simulink library "CommercialVehicleLibrary2G"  (R2021a)
settings: Solver=VariableStepAuto  StartTime=0.0  StopTime=10.0  RelTol=1e-3
values from neighbouring files (symbols this model uses):
  brake_input = [0   tmax ... (first row only)    [init_vehicle.m]    (also in run_Circle.m = [0  tmax; run_Coastdown.m = [0  2  tmax; run_DoubleLaneChangeDriver.m = [0   2  tmax; run_MaxAcc.m = [0  2  tmax)
  pose_t0 = [0 0 0 0]    [init_vehicle.m]    (also in run_Circle.m; run_Coastdown.m; run_DoubleLaneChangeDriver.m; run_MaxAcc.m)
  rdfname = 'TNO_FlatRoad.rdf'    [run_Circle.m]    (also in run_Coastdown.m; run_DoubleLaneChangeDriver.m; run_MaxAcc.m; run_Rollover.m)
  rdfname_inner = 'TNO_FlatRoad.rdf'    [run_Circle.m]    (also in run_Coastdown.m; run_DoubleLaneChangeDriver.m; run_MaxAcc.m; run_Rollover.m)
  steer_input = [0  tmax ... (first row only)    [init_vehicle.m]    (also in run_Circle.m = [0  2   10     13       tmax; run_Coastdown.m = [0 tmax; run_DoubleLaneChangeDriver.m = [0 tmax; run_MaxAcc.m = [0 tmax)
  throttle_input = [0         tmax ... (first row only)    [init_vehicle.m]    (also in run_Circle.m; run_Coastdown.m = [0        10         10.0001 tmax; run_DoubleLaneChangeDriver.m = [0        tmax; run_MaxAcc.m = [0        tmax)
  Vx = 0    [init_vehicle.m]    (also in run_Circle.m = Vx_kmh/3.6; run_Coastdown.m = Vx_kmh/3.6; run_DoubleLaneChangeDriver.m = Vx_kmh/3.6; run_MaxAcc.m)
  Vx_input = [0  tmax ... (first row only)    [init_vehicle.m]    (also in run_Circle.m; run_Coastdown.m = [0 tmax; run_DoubleLaneChangeDriver.m = [0 tmax; run_MaxAcc.m = [0 tmax)
undefined symbols (not defined in the file or in its folder): Drive, Floor, Fzstat, Fzstat1, Fzstat3, l, l_load1, l_load2, lbar, mass_load1, mass_load2, psi_semitrailer, rho, rim_Ixx, rim_Iyy, rim_mass, Steer, steer_path, tpfname, X, x_torsion, xcg, xcg1, xcg2, xcg_front, xcg_rear, xdrive1, xload1, xload2, xpos1, xref, xrev1, Xt0, Y, Yt0, Z
libraries: sm_lib x291, $bdroot x157, nesl_utility x143, vrlib x1
(part 11 of 12)

== system CommercialVehicleLibrary2G/Components/MF Tyre L/add signal names2 ==
  In1 : Inport
  Bus Creator : BusCreator  Inputs=40
  Bus Creator1 : BusCreator  Inputs=20
  Demux1 : Demux  Outputs=60
      settings: DisplayOption=none
  Terminator : Terminator
  varinf : Outport
  wires:
  Bus Creator1/1 -> Terminator/1
  Demux1/60 -> Bus Creator1/20
  Demux1/59 -> Bus Creator1/19
  Demux1/58 -> Bus Creator1/18
  Demux1/57 -> Bus Creator1/17
  Demux1/56 -> Bus Creator1/16
  Demux1/55 -> Bus Creator1/15
  Demux1/54 -> Bus Creator1/14
  Demux1/53 -> Bus Creator1/13
  Demux1/52 -> Bus Creator1/12
  Demux1/51 -> Bus Creator1/11
  Demux1/50 -> Bus Creator1/10
  Demux1/49 -> Bus Creator1/9
  Demux1/48 -> Bus Creator1/8
  Demux1/47 -> Bus Creator1/7
  Demux1/46 -> Bus Creator1/6
  Demux1/45 -> Bus Creator1/5
  Demux1/44 -> Bus Creator1/4
  Demux1/43 -> Bus Creator1/3
  Demux1/42 -> Bus Creator1/2
  Demux1/41 -> Bus Creator1/1
  Demux1/39 -> Bus Creator/39  "eff_plane_curvature"
  Demux1/38 -> Bus Creator/38  "eff_plane_angle"
  Demux1/37 -> Bus Creator/37  "eff_plane_height"
  Demux1/36 -> Bus Creator/36  "nz"
  Demux1/35 -> Bus Creator/35  "ny"
  Demux1/34 -> Bus Creator/34  "nx"
  Demux1/33 -> Bus Creator/33  "zcp"
  Demux1/32 -> Bus Creator/32  "ycp"
  Demux1/31 -> Bus Creator/31  "xcp"
  Demux1/30 -> Bus Creator/30  "_e30"
  Demux1/29 -> Bus Creator/29  "_e29"
  Demux1/28 -> Bus Creator/28  "travelled_distance"
  Demux1/27 -> Bus Creator/27  "_e27"
  Demux1/26 -> Bus Creator/26  "_e26"
  Demux1/25 -> Bus Creator/25  "_e25"
  Demux1/24 -> Bus Creator/24  "psidot"
  Demux1/23 -> Bus Creator/23  "Vz"
  Demux1/40 -> Bus Creator/40  "eff_plane_banking"
  Demux1/22 -> Bus Creator/22  "Vsy"
  Demux1/21 -> Bus Creator/21  "Vsx"
  Demux1/20 -> Bus Creator/20  "relaxation_length_y"
  Demux1/19 -> Bus Creator/19  "relaxation_length_x"
  Demux1/18 -> Bus Creator/18  "mu_y"
  Demux1/17 -> Bus Creator/17  "mu_x"
  Demux1/16 -> Bus Creator/16  "pneumatic_trail"
  Demux1/15 -> Bus Creator/15  "contact_length"
  Demux1/14 -> Bus Creator/14  "vertical_deflection"
  Demux1/13 -> Bus Creator/13  "effective_rolling_radius"
  Demux1/12 -> Bus Creator/12  "_e12"
  Demux1/11 -> Bus Creator/11  "Vx"
  Demux1/10 -> Bus Creator/10  "turn_slip"
  Demux1/9 -> Bus Creator/9  "inclination_angle"
  Demux1/8 -> Bus Creator/8  "side_slip_angle"
  Demux1/7 -> Bus Creator/7  "longitudinal_slip"
  Demux1/6 -> Bus Creator/6  "Mz"
  Demux1/5 -> Bus Creator/5  "My"
  Demux1/4 -> Bus Creator/4  "Mx"
  Demux1/3 -> Bus Creator/3  "Fz"
  Demux1/2 -> Bus Creator/2  "Fy"
  Demux1/1 -> Bus Creator/1  "Fx"
  In1/1 -> Demux1/1
  Bus Creator/1 -> varinf/1  "varinf"

== system CommercialVehicleLibrary2G/Components/MF Tyre R/add signal names2 ==
  In1 : Inport
  Bus Creator : BusCreator  Inputs=40
  Bus Creator1 : BusCreator  Inputs=20
  Demux1 : Demux  Outputs=60
      settings: DisplayOption=none
  Terminator : Terminator
  varinf : Outport
  wires:
  Bus Creator1/1 -> Terminator/1
  Demux1/60 -> Bus Creator1/20
  Demux1/59 -> Bus Creator1/19
  Demux1/58 -> Bus Creator1/18
  Demux1/57 -> Bus Creator1/17
  Demux1/56 -> Bus Creator1/16
  Demux1/55 -> Bus Creator1/15
  Demux1/54 -> Bus Creator1/14
  Demux1/53 -> Bus Creator1/13
  Demux1/52 -> Bus Creator1/12
  Demux1/51 -> Bus Creator1/11
  Demux1/50 -> Bus Creator1/10
  Demux1/49 -> Bus Creator1/9
  Demux1/48 -> Bus Creator1/8
  Demux1/47 -> Bus Creator1/7
  Demux1/46 -> Bus Creator1/6
  Demux1/45 -> Bus Creator1/5
  Demux1/44 -> Bus Creator1/4
  Demux1/43 -> Bus Creator1/3
  Demux1/42 -> Bus Creator1/2
  Demux1/41 -> Bus Creator1/1
  Demux1/39 -> Bus Creator/39  "eff_plane_curvature"
  Demux1/38 -> Bus Creator/38  "eff_plane_angle"
  Demux1/37 -> Bus Creator/37  "eff_plane_height"
  Demux1/36 -> Bus Creator/36  "nz"
  Demux1/35 -> Bus Creator/35  "ny"
  Demux1/34 -> Bus Creator/34  "nx"
  Demux1/33 -> Bus Creator/33  "zcp"
  Demux1/32 -> Bus Creator/32  "ycp"
  Demux1/31 -> Bus Creator/31  "xcp"
  Demux1/30 -> Bus Creator/30  "_e30"
  Demux1/29 -> Bus Creator/29  "_e29"
  Demux1/28 -> Bus Creator/28  "travelled_distance"
  Demux1/27 -> Bus Creator/27  "_e27"
  Demux1/26 -> Bus Creator/26  "_e26"
  Demux1/25 -> Bus Creator/25  "_e25"
  Demux1/24 -> Bus Creator/24  "psidot"
  Demux1/23 -> Bus Creator/23  "Vz"
  Demux1/40 -> Bus Creator/40  "eff_plane_banking"
  Demux1/22 -> Bus Creator/22  "Vsy"
  Demux1/21 -> Bus Creator/21  "Vsx"
  Demux1/20 -> Bus Creator/20  "relaxation_length_y"
  Demux1/19 -> Bus Creator/19  "relaxation_length_x"
  Demux1/18 -> Bus Creator/18  "mu_y"
  Demux1/17 -> Bus Creator/17  "mu_x"
  Demux1/16 -> Bus Creator/16  "pneumatic_trail"
  Demux1/15 -> Bus Creator/15  "contact_length"
  Demux1/14 -> Bus Creator/14  "vertical_deflection"
  Demux1/13 -> Bus Creator/13  "effective_rolling_radius"
  Demux1/12 -> Bus Creator/12  "_e12"
  Demux1/11 -> Bus Creator/11  "Vx"
  Demux1/10 -> Bus Creator/10  "turn_slip"
  Demux1/9 -> Bus Creator/9  "inclination_angle"
  Demux1/8 -> Bus Creator/8  "side_slip_angle"
  Demux1/7 -> Bus Creator/7  "longitudinal_slip"
  Demux1/6 -> Bus Creator/6  "Mz"
  Demux1/5 -> Bus Creator/5  "My"
  Demux1/4 -> Bus Creator/4  "Mx"
  Demux1/3 -> Bus Creator/3  "Fz"
  Demux1/2 -> Bus Creator/2  "Fy"
  Demux1/1 -> Bus Creator/1  "Fx"
  In1/1 -> Demux1/1
  Bus Creator/1 -> varinf/1  "varinf"

== system CommercialVehicleLibrary2G/Trailers/Semitrailer/Cameras ==
  Spherical Solid : sm_lib/Body Elements/Spherical Solid  GraphicAmbientColor=[0.15 0.15 0.15 1.0]  BasedOnType=Density  CenterOfMass=[0 0 0]  CenterOfMassUnits=m  GraphicDiffuseColor=[0.5 0.5 0.5]  Density=1000  DensityUnits=kg/m^3  DoExposeReferenceFrame=on  GraphicEmissiveColor=[0.0 0.0 0.0 1.0]  ExportEntireGeometry=off  SerializedExposedGeometries=<ExposedGeometries/>  SerializedFrames=<Frames/>  MarkerShape=Sphere  MarkerSize=10  GraphicType=FromGeometry  InertiaType=PointMass  Mass=1e-10  MassUnits=kg  MomentsOfInertia=[1 1 1]  MomentsOfInertiaUnits=kg*m^2  GraphicOpacity=0  ProductsOfInertia=[0 0 0]  ProductsOfInertiaUnits=kg*m^2  GraphicShininess=75  GraphicSpecularColor=[0.5 0.5 0.5 1.0]  SphereRadius=1e-10  SphereRadiusUnits=m  GraphicVisPropType=SimpleVisualProperties
  Trailer Camera Position : sm_lib/Frames and Transforms/Rigid Transform  TranslationMethod=Cartesian  TranslationStandardOffset=0  TranslationLengthUnit=m  TranslationStandardAxis=+Z  TranslationCartesianOffset=[-20 0 8]  TranslationROffset=0  TranslationROffsetUnits=m  TranslationZOffset=0  TranslationZOffsetUnits=m  TranslationThetaOffset=0  TranslationThetaOffsetUnits=deg  RotationMethod=None  RotationAngleUnits=deg  RotationStandardAxis=+Z  RotationAngle=0.0  RotationArbitraryAxis=[0 0 1]  FollAlignAxisA=+X  BaseAlignAxisA=+Y  FollAlignAxisB=+Y  BaseAlignAxisB=+Z  RotationSequenceAxes=FollowerAxes  RotationSequence=XYX  RotationSequenceAngles=[0 0 0]  RotationSequenceAnglesUnits=deg  RotationMatrix=[1 0 0; 0 1 0; 0 0 1]
  " " : PMIOPort  Side=Right
  connections:
  Spherical Solid/RConn1 -- Trailer Camera Position/RConn1
  Trailer Camera Position/LConn1 -- " "/RConn1

== system CommercialVehicleLibrary2G/Trailers/Trailer - 2 axle /Cameras ==
  Spherical Solid : sm_lib/Body Elements/Spherical Solid  GraphicAmbientColor=[0.15 0.15 0.15 1.0]  BasedOnType=Density  CenterOfMass=[0 0 0]  CenterOfMassUnits=m  GraphicDiffuseColor=[0.5 0.5 0.5]  Density=1000  DensityUnits=kg/m^3  DoExposeReferenceFrame=on  GraphicEmissiveColor=[0.0 0.0 0.0 1.0]  ExportEntireGeometry=off  SerializedExposedGeometries=<ExposedGeometries/>  SerializedFrames=<Frames/>  MarkerShape=Sphere  MarkerSize=10  GraphicType=FromGeometry  InertiaType=PointMass  Mass=1e-10  MassUnits=kg  MomentsOfInertia=[1 1 1]  MomentsOfInertiaUnits=kg*m^2  GraphicOpacity=0  ProductsOfInertia=[0 0 0]  ProductsOfInertiaUnits=kg*m^2  GraphicShininess=75  GraphicSpecularColor=[0.5 0.5 0.5 1.0]  SphereRadius=1e-10  SphereRadiusUnits=m  GraphicVisPropType=SimpleVisualProperties
  Trailer Camera Position : sm_lib/Frames and Transforms/Rigid Transform  TranslationMethod=Cartesian  TranslationStandardOffset=0  TranslationLengthUnit=m  TranslationStandardAxis=+Z  TranslationCartesianOffset=[-20 0 8]  TranslationROffset=0  TranslationROffsetUnits=m  TranslationZOffset=0  TranslationZOffsetUnits=m  TranslationThetaOffset=0  TranslationThetaOffsetUnits=deg  RotationMethod=None  RotationAngleUnits=deg  RotationStandardAxis=+Z  RotationAngle=0.0  RotationArbitraryAxis=[0 0 1]  FollAlignAxisA=+X  BaseAlignAxisA=+Y  FollAlignAxisB=+Y  BaseAlignAxisB=+Z  RotationSequenceAxes=FollowerAxes  RotationSequence=XYX  RotationSequenceAngles=[0 0 0]  RotationSequenceAnglesUnits=deg  RotationMatrix=[1 0 0; 0 1 0; 0 0 1]
  " " : PMIOPort  Side=Right
  connections:
  Spherical Solid/RConn1 -- Trailer Camera Position/RConn1
  Trailer Camera Position/LConn1 -- " "/RConn1

== system CommercialVehicleLibrary2G/Trailers/Trailer - 3 axle /Cameras ==
  Spherical Solid : sm_lib/Body Elements/Spherical Solid  GraphicAmbientColor=[0.15 0.15 0.15 1.0]  BasedOnType=Density  CenterOfMass=[0 0 0]  CenterOfMassUnits=m  GraphicDiffuseColor=[0.5 0.5 0.5]  Density=1000  DensityUnits=kg/m^3  DoExposeReferenceFrame=on  GraphicEmissiveColor=[0.0 0.0 0.0 1.0]  ExportEntireGeometry=off  SerializedExposedGeometries=<ExposedGeometries/>  SerializedFrames=<Frames/>  MarkerShape=Sphere  MarkerSize=10  GraphicType=FromGeometry  InertiaType=PointMass  Mass=1e-10  MassUnits=kg  MomentsOfInertia=[1 1 1]  MomentsOfInertiaUnits=kg*m^2  GraphicOpacity=0  ProductsOfInertia=[0 0 0]  ProductsOfInertiaUnits=kg*m^2  GraphicShininess=75  GraphicSpecularColor=[0.5 0.5 0.5 1.0]  SphereRadius=1e-10  SphereRadiusUnits=m  GraphicVisPropType=SimpleVisualProperties
  Trailer Camera Position : sm_lib/Frames and Transforms/Rigid Transform  TranslationMethod=Cartesian  TranslationStandardOffset=0  TranslationLengthUnit=m  TranslationStandardAxis=+Z  TranslationCartesianOffset=[-20 0 8]  TranslationROffset=0  TranslationROffsetUnits=m  TranslationZOffset=0  TranslationZOffsetUnits=m  TranslationThetaOffset=0  TranslationThetaOffsetUnits=deg  RotationMethod=None  RotationAngleUnits=deg  RotationStandardAxis=+Z  RotationAngle=0.0  RotationArbitraryAxis=[0 0 1]  FollAlignAxisA=+X  BaseAlignAxisA=+Y  FollAlignAxisB=+Y  BaseAlignAxisB=+Z  RotationSequenceAxes=FollowerAxes  RotationSequence=XYX  RotationSequenceAngles=[0 0 0]  RotationSequenceAnglesUnits=deg  RotationMatrix=[1 0 0; 0 1 0; 0 0 1]
  " " : PMIOPort  Side=Right
  connections:
  Spherical Solid/RConn1 -- Trailer Camera Position/RConn1
  Trailer Camera Position/LConn1 -- " "/RConn1

== system CommercialVehicleLibrary2G/Utilities/To_workspace_dolly/Subsystem ==
  In1 : Inport
  Bus Selector24 : BusSelector  OutputSignals=axle1.Tire_L.Fx,axle1.Tire_R.Fx,axle2.Tire_L.Fx,axle2.Tire_R.Fx
  Mux : Mux
  Out1 : Outport
  wires:
  Bus Selector24/4 -> Mux/4  "<Fx>"
  Bus Selector24/3 -> Mux/3  "<Fx>"
  Bus Selector24/2 -> Mux/2  "<Fx>"
  Bus Selector24/1 -> Mux/1  "<Fx>"
  Mux/1 -> Out1/1
  In1/1 -> Bus Selector24/1

== system CommercialVehicleLibrary2G/Utilities/To_workspace_dolly/Subsystem1 ==
  In1 : Inport
  Bus Selector24 : BusSelector  OutputSignals=axle1.Tire_L.Fy,axle1.Tire_R.Fy,axle2.Tire_L.Fy,axle2.Tire_R.Fy
  Mux : Mux
  Out1 : Outport
  wires:
  Mux/1 -> Out1/1
  In1/1 -> Bus Selector24/1
  Bus Selector24/1 -> Mux/1  "<Fy>"
  Bus Selector24/2 -> Mux/2  "<Fy>"
  Bus Selector24/3 -> Mux/3  "<Fy>"
  Bus Selector24/4 -> Mux/4  "<Fy>"

== system CommercialVehicleLibrary2G/Utilities/To_workspace_dolly/Subsystem2 ==
  In1 : Inport
  Bus Selector24 : BusSelector  OutputSignals=axle1.Tire_L.Fz,axle1.Tire_R.Fz,axle2.Tire_L.Fz,axle2.Tire_R.Fz
  Mux : Mux
  Out1 : Outport
  wires:
  Mux/1 -> Out1/1
  In1/1 -> Bus Selector24/1
  Bus Selector24/1 -> Mux/1  "<Fz>"
  Bus Selector24/2 -> Mux/2  "<Fz>"
  Bus Selector24/3 -> Mux/3  "<Fz>"
  Bus Selector24/4 -> Mux/4  "<Fz>"

== system CommercialVehicleLibrary2G/Utilities/To_workspace_dolly/Subsystem3 ==
  In1 : Inport
  Bus Selector6 : BusSelector  OutputSignals=axle1.Omega1,axle1.Omega2,axle2.Omega1,axle2.Omega2
  Mux : Mux
  Out1 : Outport
  wires:
  In1/1 -> Bus Selector6/1
  Mux/1 -> Out1/1
  Bus Selector6/1 -> Mux/1  "<Omega1>"
  Bus Selector6/2 -> Mux/2  "<Omega2>"
  Bus Selector6/3 -> Mux/3  "<Omega1>"
  Bus Selector6/4 -> Mux/4  "<Omega2>"

== system CommercialVehicleLibrary2G/Utilities/To_workspace_drawbar_trailer_2axle/Subsystem ==
  In1 : Inport
  Bus Selector24 : BusSelector  OutputSignals=axle1.Tire_L.Fx,axle1.Tire_R.Fx,axle2.Tire_L.Fx,axle2.Tire_R.Fx
  Mux : Mux
  Out1 : Outport
  wires:
  Bus Selector24/4 -> Mux/4  "<Fx>"
  Bus Selector24/3 -> Mux/3  "<Fx>"
  Bus Selector24/2 -> Mux/2  "<Fx>"
  Bus Selector24/1 -> Mux/1  "<Fx>"
  Mux/1 -> Out1/1
  In1/1 -> Bus Selector24/1

== system CommercialVehicleLibrary2G/Utilities/To_workspace_drawbar_trailer_2axle/Subsystem1 ==
  In1 : Inport
  Bus Selector24 : BusSelector  OutputSignals=axle1.Tire_L.Fy,axle1.Tire_R.Fy,axle2.Tire_L.Fy,axle2.Tire_R.Fy
  Mux : Mux
  Out1 : Outport
  wires:
  Mux/1 -> Out1/1
  In1/1 -> Bus Selector24/1
  Bus Selector24/1 -> Mux/1  "<Fy>"
  Bus Selector24/2 -> Mux/2  "<Fy>"
  Bus Selector24/3 -> Mux/3  "<Fy>"
  Bus Selector24/4 -> Mux/4  "<Fy>"

== system CommercialVehicleLibrary2G/Utilities/To_workspace_drawbar_trailer_2axle/Subsystem2 ==
  In1 : Inport
  Bus Selector24 : BusSelector  OutputSignals=axle1.Tire_L.Fz,axle1.Tire_R.Fz,axle2.Tire_L.Fz,axle2.Tire_R.Fz
  Mux : Mux
  Out1 : Outport
  wires:
  Mux/1 -> Out1/1
  In1/1 -> Bus Selector24/1
  Bus Selector24/1 -> Mux/1  "<Fz>"
  Bus Selector24/2 -> Mux/2  "<Fz>"
  Bus Selector24/3 -> Mux/3  "<Fz>"
  Bus Selector24/4 -> Mux/4  "<Fz>"

== system CommercialVehicleLibrary2G/Utilities/To_workspace_drawbar_trailer_2axle/Subsystem3 ==
  In1 : Inport
  Bus Selector6 : BusSelector  OutputSignals=axle1.Omega1,axle1.Omega2,axle2.Omega1,axle2.Omega2
  Mux : Mux
  Out1 : Outport
  wires:
  In1/1 -> Bus Selector6/1
  Mux/1 -> Out1/1
  Bus Selector6/1 -> Mux/1  "<Omega1>"
  Bus Selector6/2 -> Mux/2  "<Omega2>"
  Bus Selector6/3 -> Mux/3  "<Omega1>"
  Bus Selector6/4 -> Mux/4  "<Omega2>"

== system CommercialVehicleLibrary2G/Utilities/To_workspace_drawbar_trailer_3axle/Subsystem ==
  In1 : Inport
  Bus Selector24 : BusSelector  OutputSignals=axle1.Tire_L.Fx,axle1.Tire_R.Fx,axle2.Tire_L.Fx,axle2.Tire_R.Fx
  Mux : Mux
  Out1 : Outport
  wires:
  Bus Selector24/4 -> Mux/4  "<Fx>"
  Bus Selector24/3 -> Mux/3  "<Fx>"
  Bus Selector24/2 -> Mux/2  "<Fx>"
  Bus Selector24/1 -> Mux/1  "<Fx>"
  Mux/1 -> Out1/1
  In1/1 -> Bus Selector24/1

== system CommercialVehicleLibrary2G/Utilities/To_workspace_drawbar_trailer_3axle/Subsystem1 ==
  In1 : Inport
  Bus Selector24 : BusSelector  OutputSignals=axle1.Tire_L.Fy,axle1.Tire_R.Fy,axle2.Tire_L.Fy,axle2.Tire_R.Fy
  Mux : Mux
  Out1 : Outport
  wires:
  Mux/1 -> Out1/1
  In1/1 -> Bus Selector24/1
  Bus Selector24/1 -> Mux/1  "<Fy>"
  Bus Selector24/2 -> Mux/2  "<Fy>"
  Bus Selector24/3 -> Mux/3  "<Fy>"
  Bus Selector24/4 -> Mux/4  "<Fy>"

== system CommercialVehicleLibrary2G/Utilities/To_workspace_drawbar_trailer_3axle/Subsystem2 ==
  In1 : Inport
  Bus Selector24 : BusSelector  OutputSignals=axle1.Tire_L.Fz,axle1.Tire_R.Fz,axle2.Tire_L.Fz,axle2.Tire_R.Fz
  Mux : Mux
  Out1 : Outport
  wires:
  Mux/1 -> Out1/1
  In1/1 -> Bus Selector24/1
  Bus Selector24/1 -> Mux/1  "<Fz>"
  Bus Selector24/2 -> Mux/2  "<Fz>"
  Bus Selector24/3 -> Mux/3  "<Fz>"
  Bus Selector24/4 -> Mux/4  "<Fz>"

== system CommercialVehicleLibrary2G/Utilities/To_workspace_drawbar_trailer_3axle/Subsystem3 ==
  In1 : Inport
  Bus Selector6 : BusSelector  OutputSignals=axle1.Omega1,axle1.Omega2,axle2.Omega1,axle2.Omega2
  Mux : Mux
  Out1 : Outport
  wires:
  In1/1 -> Bus Selector6/1
  Mux/1 -> Out1/1
  Bus Selector6/1 -> Mux/1  "<Omega1>"
  Bus Selector6/2 -> Mux/2  "<Omega2>"
  Bus Selector6/3 -> Mux/3  "<Omega1>"
  Bus Selector6/4 -> Mux/4  "<Omega2>"

== system CommercialVehicleLibrary2G/Utilities/To_workspace_semitrailer/Subsystem ==
  In1 : Inport
  Bus Selector24 : BusSelector  OutputSignals=axle1.Tire_L.Fx,axle1.Tire_R.Fx,axle2.Tire_L.Fx,axle2.Tire_R.Fx,axle3.Tire_L.Fx,axle3.Tire_R.Fx
  Mux : Mux  Inputs=6
  Out1 : Outport
  wires:
  Bus Selector24/4 -> Mux/4  "<Fx>"
  Bus Selector24/3 -> Mux/3  "<Fx>"
  Bus Selector24/2 -> Mux/2  "<Fx>"
  Bus Selector24/1 -> Mux/1  "<Fx>"
  Mux/1 -> Out1/1
  In1/1 -> Bus Selector24/1
  Bus Selector24/5 -> Mux/5  "<Fx>"
  Bus Selector24/6 -> Mux/6  "<Fx>"

== system CommercialVehicleLibrary2G/Utilities/To_workspace_semitrailer/Subsystem1 ==
  In1 : Inport
  Bus Selector24 : BusSelector  OutputSignals=axle1.Tire_L.Fy,axle1.Tire_R.Fy,axle2.Tire_L.Fy,axle2.Tire_R.Fy,axle3.Tire_L.Fy,axle3.Tire_R.Fy
  Mux : Mux  Inputs=6
  Out1 : Outport
  wires:
  Mux/1 -> Out1/1
  In1/1 -> Bus Selector24/1
  Bus Selector24/1 -> Mux/1  "<Fy>"
  Bus Selector24/2 -> Mux/2  "<Fy>"
  Bus Selector24/3 -> Mux/3  "<Fy>"
  Bus Selector24/4 -> Mux/4  "<Fy>"
  Bus Selector24/5 -> Mux/5  "<Fy>"
  Bus Selector24/6 -> Mux/6  "<Fy>"

== system CommercialVehicleLibrary2G/Utilities/To_workspace_semitrailer/Subsystem2 ==
  In1 : Inport
  Bus Selector24 : BusSelector  OutputSignals=axle1.Tire_L.Fz,axle1.Tire_R.Fz,axle2.Tire_L.Fz,axle2.Tire_R.Fz,axle3.Tire_L.Fz,axle3.Tire_R.Fz
  Mux : Mux  Inputs=6
  Out1 : Outport
  wires:
  Mux/1 -> Out1/1
  In1/1 -> Bus Selector24/1
  Bus Selector24/1 -> Mux/1  "<Fz>"
  Bus Selector24/2 -> Mux/2  "<Fz>"
  Bus Selector24/3 -> Mux/3  "<Fz>"
  Bus Selector24/4 -> Mux/4  "<Fz>"
  Bus Selector24/5 -> Mux/5  "<Fz>"
  Bus Selector24/6 -> Mux/6  "<Fz>"

== system CommercialVehicleLibrary2G/Utilities/To_workspace_semitrailer/Subsystem3 ==
  In1 : Inport
  Bus Selector6 : BusSelector  OutputSignals=axle1.Omega1,axle1.Omega2,axle2.Omega1,axle2.Omega2,axle3.Omega1,axle3.Omega2
  Mux : Mux  Inputs=6
  Out1 : Outport
  wires:
  In1/1 -> Bus Selector6/1
  Mux/1 -> Out1/1
  Bus Selector6/1 -> Mux/1  "<Omega1>"
  Bus Selector6/2 -> Mux/2  "<Omega2>"
  Bus Selector6/3 -> Mux/3  "<Omega1>"
  Bus Selector6/4 -> Mux/4  "<Omega2>"
  Bus Selector6/5 -> Mux/5  "<Omega1>"
  Bus Selector6/6 -> Mux/6  "<Omega2>"

== system CommercialVehicleLibrary2G/Utilities/To_workspace_tractor/Subsystem ==
  In1 : Inport
  Bus Selector24 : BusSelector  OutputSignals=steeraxle.Tire1_L.Fx,steeraxle.Tire1_R.Fx,driveaxle.Tire1_L.Fx,driveaxle.Tire2_L.Fx,driveaxle.Tire1_R.Fx,driveaxle.Tire2_R.Fx
  Mux : Mux  Inputs=6
  Out1 : Outport
  wires:
  Bus Selector24/6 -> Mux/6  "<Fx>"
  Bus Selector24/5 -> Mux/5  "<Fx>"
  Bus Selector24/4 -> Mux/4  "<Fx>"
  Bus Selector24/3 -> Mux/3  "<Fx>"
  Bus Selector24/2 -> Mux/2  "<Fx>"
  Bus Selector24/1 -> Mux/1  "<Fx>"
  Mux/1 -> Out1/1
  In1/1 -> Bus Selector24/1

== system CommercialVehicleLibrary2G/Utilities/To_workspace_tractor/Subsystem1 ==
  In1 : Inport
  Bus Selector24 : BusSelector  OutputSignals=steeraxle.Tire1_L.Fy,steeraxle.Tire1_R.Fy,driveaxle.Tire1_L.Fy,driveaxle.Tire2_L.Fy,driveaxle.Tire1_R.Fy,driveaxle.Tire2_R.Fy
  Mux : Mux  Inputs=6
  Out1 : Outport
  wires:
  Bus Selector24/6 -> Mux/6  "<Fy>"
  Bus Selector24/5 -> Mux/5  "<Fy>"
  Bus Selector24/4 -> Mux/4  "<Fy>"
  Bus Selector24/3 -> Mux/3  "<Fy>"
  Bus Selector24/2 -> Mux/2  "<Fy>"
  Bus Selector24/1 -> Mux/1  "<Fy>"
  Mux/1 -> Out1/1
  In1/1 -> Bus Selector24/1

== system CommercialVehicleLibrary2G/Utilities/To_workspace_tractor/Subsystem2 ==
  In1 : Inport
  Bus Selector24 : BusSelector  OutputSignals=steeraxle.Tire1_L.Fz,steeraxle.Tire1_R.Fz,driveaxle.Tire1_L.Fz,driveaxle.Tire2_L.Fz,driveaxle.Tire1_R.Fz,driveaxle.Tire2_R.Fz
  Mux : Mux  Inputs=6
  Out1 : Outport
  wires:
  Bus Selector24/6 -> Mux/6  "<Fz>"
  Bus Selector24/5 -> Mux/5  "<Fz>"
  Bus Selector24/4 -> Mux/4  "<Fz>"
  Bus Selector24/3 -> Mux/3  "<Fz>"
  Bus Selector24/2 -> Mux/2  "<Fz>"
  Bus Selector24/1 -> Mux/1  "<Fz>"
  Mux/1 -> Out1/1
  In1/1 -> Bus Selector24/1

== system CommercialVehicleLibrary2G/Utilities/To_workspace_tractor/Subsystem3 ==
  In1 : Inport
  Bus Selector6 : BusSelector  OutputSignals=steeraxle.Omega1,steeraxle.Omega2,driveaxle.Omega1,driveaxle.Omega2
  Mux : Mux
  Out1 : Outport
  wires:
  In1/1 -> Bus Selector6/1
  Mux/1 -> Out1/1
  Bus Selector6/1 -> Mux/1  "<Omega1>"
  Bus Selector6/3 -> Mux/3  "<Omega1>"
  Bus Selector6/4 -> Mux/4  "<Omega2>"
  Bus Selector6/2 -> Mux/2  "<Omega2>"

== system CommercialVehicleLibrary2G/Utilities/To_workspace_trailer_2axle/Subsystem ==
  In1 : Inport
  Bus Selector24 : BusSelector  OutputSignals=axle1.Tire_L.Fx,axle1.Tire_R.Fx,axle2.Tire_L.Fx,axle2.Tire_R.Fx
  Mux : Mux
  Out1 : Outport
  wires:
  Bus Selector24/4 -> Mux/4  "<Fx>"
  Bus Selector24/3 -> Mux/3  "<Fx>"
  Bus Selector24/2 -> Mux/2  "<Fx>"
  Bus Selector24/1 -> Mux/1  "<Fx>"
  Mux/1 -> Out1/1
  In1/1 -> Bus Selector24/1

== system CommercialVehicleLibrary2G/Utilities/To_workspace_trailer_2axle/Subsystem1 ==
  In1 : Inport
  Bus Selector24 : BusSelector  OutputSignals=axle1.Tire_L.Fy,axle1.Tire_R.Fy,axle2.Tire_L.Fy,axle2.Tire_R.Fy
  Mux : Mux
  Out1 : Outport
  wires:
  Mux/1 -> Out1/1
  In1/1 -> Bus Selector24/1
  Bus Selector24/1 -> Mux/1  "<Fy>"
  Bus Selector24/2 -> Mux/2  "<Fy>"
  Bus Selector24/3 -> Mux/3  "<Fy>"
  Bus Selector24/4 -> Mux/4  "<Fy>"

== system CommercialVehicleLibrary2G/Utilities/To_workspace_trailer_2axle/Subsystem2 ==
  In1 : Inport
  Bus Selector24 : BusSelector  OutputSignals=axle1.Tire_L.Fz,axle1.Tire_R.Fz,axle2.Tire_L.Fz,axle2.Tire_R.Fz
  Mux : Mux
  Out1 : Outport
  wires:
  Mux/1 -> Out1/1
  In1/1 -> Bus Selector24/1
  Bus Selector24/1 -> Mux/1  "<Fz>"
  Bus Selector24/2 -> Mux/2  "<Fz>"
  Bus Selector24/3 -> Mux/3  "<Fz>"
  Bus Selector24/4 -> Mux/4  "<Fz>"

== system CommercialVehicleLibrary2G/Utilities/To_workspace_trailer_2axle/Subsystem3 ==
  In1 : Inport
  Bus Selector6 : BusSelector  OutputSignals=axle1.Omega1,axle1.Omega2,axle2.Omega1,axle2.Omega2
  Mux : Mux
  Out1 : Outport
  wires:
  In1/1 -> Bus Selector6/1
  Mux/1 -> Out1/1
  Bus Selector6/1 -> Mux/1  "<Omega1>"
  Bus Selector6/2 -> Mux/2  "<Omega2>"
  Bus Selector6/3 -> Mux/3  "<Omega1>"
  Bus Selector6/4 -> Mux/4  "<Omega2>"

== system CommercialVehicleLibrary2G/Utilities/To_workspace_trailer_3axle/Subsystem ==
  In1 : Inport
  Bus Selector24 : BusSelector  OutputSignals=axle1.Tire_L.Fx,axle1.Tire_R.Fx,axle2.Tire_L.Fx,axle2.Tire_R.Fx
  Mux : Mux
  Out1 : Outport
  wires:
  Bus Selector24/4 -> Mux/4  "<Fx>"
  Bus Selector24/3 -> Mux/3  "<Fx>"
  Bus Selector24/2 -> Mux/2  "<Fx>"
  Bus Selector24/1 -> Mux/1  "<Fx>"
  Mux/1 -> Out1/1
  In1/1 -> Bus Selector24/1

== system CommercialVehicleLibrary2G/Utilities/To_workspace_trailer_3axle/Subsystem1 ==
  In1 : Inport
  Bus Selector24 : BusSelector  OutputSignals=axle1.Tire_L.Fy,axle1.Tire_R.Fy,axle2.Tire_L.Fy,axle2.Tire_R.Fy
  Mux : Mux
  Out1 : Outport
  wires:
  Mux/1 -> Out1/1
  In1/1 -> Bus Selector24/1
  Bus Selector24/1 -> Mux/1  "<Fy>"
  Bus Selector24/2 -> Mux/2  "<Fy>"
  Bus Selector24/3 -> Mux/3  "<Fy>"
  Bus Selector24/4 -> Mux/4  "<Fy>"

== system CommercialVehicleLibrary2G/Utilities/To_workspace_trailer_3axle/Subsystem2 ==
  In1 : Inport
  Bus Selector24 : BusSelector  OutputSignals=axle1.Tire_L.Fz,axle1.Tire_R.Fz,axle2.Tire_L.Fz,axle2.Tire_R.Fz
  Mux : Mux
  Out1 : Outport
  wires:
  Mux/1 -> Out1/1
  In1/1 -> Bus Selector24/1
  Bus Selector24/1 -> Mux/1  "<Fz>"
  Bus Selector24/2 -> Mux/2  "<Fz>"
  Bus Selector24/3 -> Mux/3  "<Fz>"
  Bus Selector24/4 -> Mux/4  "<Fz>"

== system CommercialVehicleLibrary2G/Utilities/To_workspace_trailer_3axle/Subsystem3 ==
  In1 : Inport
  Bus Selector6 : BusSelector  OutputSignals=axle1.Omega1,axle1.Omega2,axle2.Omega1,axle2.Omega2
  Mux : Mux
  Out1 : Outport
  wires:
  In1/1 -> Bus Selector6/1
  Mux/1 -> Out1/1
  Bus Selector6/1 -> Mux/1  "<Omega1>"
  Bus Selector6/2 -> Mux/2  "<Omega2>"
  Bus Selector6/3 -> Mux/3  "<Omega1>"
  Bus Selector6/4 -> Mux/4  "<Omega2>"

== system CommercialVehicleLibrary2G/Utilities/To_workspace_truck_2axle/Subsystem ==
  In1 : Inport
  Bus Selector24 : BusSelector  OutputSignals=steeraxle.Tire1_L.Fx,steeraxle.Tire1_R.Fx,driveaxle.Tire1_L.Fx,driveaxle.Tire2_L.Fx,driveaxle.Tire1_R.Fx,driveaxle.Tire2_R.Fx
  Mux : Mux  Inputs=6
  Out1 : Outport
  wires:
  In1/1 -> Bus Selector24/1
  Mux/1 -> Out1/1
  Bus Selector24/1 -> Mux/1  "<Fx>"
  Bus Selector24/2 -> Mux/2  "<Fx>"
  Bus Selector24/3 -> Mux/3  "<Fx>"
  Bus Selector24/4 -> Mux/4  "<Fx>"
  Bus Selector24/5 -> Mux/5  "<Fx>"
  Bus Selector24/6 -> Mux/6  "<Fx>"

== system CommercialVehicleLibrary2G/Utilities/To_workspace_truck_2axle/Subsystem1 ==
  In1 : Inport
  Bus Selector24 : BusSelector  OutputSignals=steeraxle.Tire1_L.Fy,steeraxle.Tire1_R.Fy,driveaxle.Tire1_L.Fy,driveaxle.Tire2_L.Fy,driveaxle.Tire1_R.Fy,driveaxle.Tire2_R.Fy
  Mux : Mux  Inputs=6
  Out1 : Outport
  wires:
  In1/1 -> Bus Selector24/1
  Mux/1 -> Out1/1
  Bus Selector24/1 -> Mux/1  "<Fy>"
  Bus Selector24/2 -> Mux/2  "<Fy>"
  Bus Selector24/3 -> Mux/3  "<Fy>"
  Bus Selector24/4 -> Mux/4  "<Fy>"
  Bus Selector24/5 -> Mux/5  "<Fy>"
  Bus Selector24/6 -> Mux/6  "<Fy>"

== system CommercialVehicleLibrary2G/Utilities/To_workspace_truck_2axle/Subsystem2 ==
  In1 : Inport
  Bus Selector24 : BusSelector  OutputSignals=steeraxle.Tire1_L.Fz,steeraxle.Tire1_R.Fz,driveaxle.Tire1_L.Fz,driveaxle.Tire2_L.Fz,driveaxle.Tire1_R.Fz,driveaxle.Tire2_R.Fz
  Mux : Mux  Inputs=6
  Out1 : Outport
  wires:
  In1/1 -> Bus Selector24/1
  Mux/1 -> Out1/1
  Bus Selector24/1 -> Mux/1  "<Fz>"
  Bus Selector24/2 -> Mux/2  "<Fz>"
  Bus Selector24/3 -> Mux/3  "<Fz>"
  Bus Selector24/4 -> Mux/4  "<Fz>"
  Bus Selector24/5 -> Mux/5  "<Fz>"
  Bus Selector24/6 -> Mux/6  "<Fz>"

== system CommercialVehicleLibrary2G/Utilities/To_workspace_truck_2axle/Subsystem3 ==
  In1 : Inport
  Bus Selector6 : BusSelector  OutputSignals=steeraxle.Omega1,steeraxle.Omega2,driveaxle.Omega1,driveaxle.Omega2
  Mux : Mux
  Out1 : Outport
  wires:
  Bus Selector6/2 -> Mux/2  "<Omega2>"
  Bus Selector6/4 -> Mux/4  "<Omega2>"
  Bus Selector6/3 -> Mux/3  "<Omega1>"
  Bus Selector6/1 -> Mux/1  "<Omega1>"
  Mux/1 -> Out1/1
  In1/1 -> Bus Selector6/1

== system CommercialVehicleLibrary2G/Utilities/To_workspace_truck_3axle/Subsystem ==
  In1 : Inport
  Bus Selector24 : BusSelector  OutputSignals=steeraxle.Tyre1(L).Fx,steeraxle.Tyre1(R).Fx,driveaxle1.G2_Tire 1 RL.Fx,driveaxle1.G2_Tire 2 RL.Fx,driveaxle1.G2_Tire 1 RR.Fx,driveaxle1.G2_Tire 2 RR.Fx
  Mux : Mux  Inputs=6
  Out1 : Outport
  wires:
  In1/1 -> Bus Selector24/1
  Mux/1 -> Out1/1
  Bus Selector24/1 -> Mux/1  "<Fx>"
  Bus Selector24/2 -> Mux/2  "<Fx>"
  Bus Selector24/3 -> Mux/3  "<Fx>"
  Bus Selector24/4 -> Mux/4  "<Fx>"
  Bus Selector24/5 -> Mux/5  "<Fx>"
  Bus Selector24/6 -> Mux/6  "<Fx>"

== system CommercialVehicleLibrary2G/Utilities/To_workspace_truck_3axle/Subsystem1 ==
  In1 : Inport
  Bus Selector24 : BusSelector  OutputSignals=steeraxle.Tyre1(L).Fy,steeraxle.Tyre1(R).Fy,driveaxle1.G2_Tire 1 RL.Fy,driveaxle1.G2_Tire 2 RL.Fy,driveaxle1.G2_Tire 1 RR.Fy,driveaxle1.G2_Tire 2 RR.Fy
  Mux : Mux  Inputs=6
  Out1 : Outport
  wires:
  In1/1 -> Bus Selector24/1
  Mux/1 -> Out1/1
  Bus Selector24/1 -> Mux/1  "<Fy>"
  Bus Selector24/2 -> Mux/2  "<Fy>"
  Bus Selector24/3 -> Mux/3  "<Fy>"
  Bus Selector24/4 -> Mux/4  "<Fy>"
  Bus Selector24/5 -> Mux/5  "<Fy>"
  Bus Selector24/6 -> Mux/6  "<Fy>"

== system CommercialVehicleLibrary2G/Utilities/To_workspace_truck_3axle/Subsystem3 ==
  In1 : Inport
  Bus Selector6 : BusSelector  OutputSignals=steeraxle.Omega1 (LF),steeraxle.Omega2 (RF),driveaxle1.G2_omega1_Tire1-2(RL),driveaxle1.G2_omega2_Tire1-2(RR)
  Mux : Mux
  Out1 : Outport
  wires:
  Bus Selector6/2 -> Mux/2  "<Omega2 (RF)>"
  Bus Selector6/4 -> Mux/4  "<G2_omega2_Tire1-2(RR)>"
  Bus Selector6/3 -> Mux/3  "<G2_omega1_Tire1-2(RL)>"
  Bus Selector6/1 -> Mux/1  "<Omega1 (LF)>"
  Mux/1 -> Out1/1
  In1/1 -> Bus Selector6/1

== system CommercialVehicleLibrary2G/Utilities/To_workspace_truck_3axle/Subsystem4 ==
  In1 : Inport
  Bus Selector24 : BusSelector  OutputSignals=steeraxle.Tire1_L.Fz,steeraxle.Tire1_R.Fz,driveaxle1.Tire1_L.Fz,driveaxle1.Tire2_L.Fz,driveaxle1.Tire1_R.Fz,driveaxle1.Tire2_R.Fz,driveaxle2.Tire1_L.Fz,driveaxle2.Tire2_L.Fz,driveaxle2.Tire1_R.Fz,driveaxle2.Tire2_R.Fz
  Mux : Mux  Inputs=10
  Out1 : Outport
  wires:
  In1/1 -> Bus Selector24/1
  Mux/1 -> Out1/1
  Bus Selector24/1 -> Mux/1  "<Fz>"
  Bus Selector24/2 -> Mux/2  "<Fz>"
  Bus Selector24/3 -> Mux/3  "<Fz>"
  Bus Selector24/4 -> Mux/4  "<Fz>"
  Bus Selector24/5 -> Mux/5  "<Fz>"
  Bus Selector24/6 -> Mux/6  "<Fz>"
  Bus Selector24/7 -> Mux/7  "<Fz>"
  Bus Selector24/8 -> Mux/8  "<Fz>"
  Bus Selector24/9 -> Mux/9  "<Fz>"
  Bus Selector24/10 -> Mux/10  "<Fz>"

== system CommercialVehicleLibrary2G/Utilities/To_workspace_truck_4axle/Subsystem ==
  In1 : Inport
  Bus Selector24 : BusSelector  OutputSignals=steeraxle1.Tire1_L.Fx,steeraxle1.Tire1_R.Fx,steeraxle2.Tire1_L.Fx,steeraxle2.Tire1_R.Fx,driveaxle1.Tire1_L.Fx,driveaxle1.Tire2_L.Fx,driveaxle1.Tire1_R.Fx,driveaxle1.Tire2_R.Fx,driveaxle2.Tire1_L.Fx,driveaxle2.Tire2_L.Fx,driveaxle2.Tire1_R.Fx,driveaxle2.Tire2_R.Fx
  Mux : Mux  Inputs=12
  Out1 : Outport
  wires:
  Bus Selector24/12 -> Mux/12  "<Fx>"
  Bus Selector24/11 -> Mux/11  "<Fx>"
  Bus Selector24/10 -> Mux/10  "<Fx>"
  Bus Selector24/9 -> Mux/9  "<Fx>"
  Bus Selector24/8 -> Mux/8  "<Fx>"
  Bus Selector24/7 -> Mux/7  "<Fx>"
  Bus Selector24/6 -> Mux/6  "<Fx>"
  Bus Selector24/5 -> Mux/5  "<Fx>"
  Bus Selector24/4 -> Mux/4  "<Fx>"
  Bus Selector24/3 -> Mux/3  "<Fx>"
  Bus Selector24/2 -> Mux/2  "<Fx>"
  Bus Selector24/1 -> Mux/1  "<Fx>"
  In1/1 -> Bus Selector24/1
  Mux/1 -> Out1/1

== system CommercialVehicleLibrary2G/Utilities/To_workspace_truck_4axle/Subsystem1 ==
  In1 : Inport
  Bus Selector24 : BusSelector  OutputSignals=steeraxle1.Tire1_L.Fy,steeraxle1.Tire1_R.Fy,steeraxle2.Tire1_L.Fy,steeraxle2.Tire1_R.Fy,driveaxle1.Tire1_L.Fy,driveaxle1.Tire2_L.Fy,driveaxle1.Tire1_R.Fy,driveaxle1.Tire2_R.Fy,driveaxle2.Tire1_L.Fy,driveaxle2.Tire2_L.Fy,driveaxle2.Tire1_R.Fy,driveaxle2.Tire2_R.Fy
  Mux : Mux  Inputs=12
  Out1 : Outport
  wires:
  Bus Selector24/12 -> Mux/12  "<Fy>"
  Bus Selector24/11 -> Mux/11  "<Fy>"
  Bus Selector24/10 -> Mux/10  "<Fy>"
  Bus Selector24/9 -> Mux/9  "<Fy>"
  Bus Selector24/8 -> Mux/8  "<Fy>"
  Bus Selector24/7 -> Mux/7  "<Fy>"
  Bus Selector24/6 -> Mux/6  "<Fy>"
  Bus Selector24/5 -> Mux/5  "<Fy>"
  Bus Selector24/4 -> Mux/4  "<Fy>"
  Bus Selector24/3 -> Mux/3  "<Fy>"
  Bus Selector24/2 -> Mux/2  "<Fy>"
  Bus Selector24/1 -> Mux/1  "<Fy>"
  In1/1 -> Bus Selector24/1
  Mux/1 -> Out1/1

== system CommercialVehicleLibrary2G/Utilities/To_workspace_truck_4axle/Subsystem3 ==
  In1 : Inport
  Bus Selector6 : BusSelector  OutputSignals=steeraxle1.Omega1,steeraxle1.Omega2,steeraxle2.Omega1,steeraxle2.Omega2,driveaxle1.Omega1,driveaxle1.Omega2,driveaxle2.Omega1,driveaxle2.Omega2
  Mux : Mux  Inputs=8
  Out1 : Outport
  wires:
  Bus Selector6/8 -> Mux/8  "<Omega2>"
  Bus Selector6/7 -> Mux/7  "<Omega1>"
  Bus Selector6/6 -> Mux/6  "<Omega2>"
  Bus Selector6/5 -> Mux/5  "<Omega1>"
  Bus Selector6/4 -> Mux/4  "<Omega2>"
  Bus Selector6/3 -> Mux/3  "<Omega1>"
  Bus Selector6/2 -> Mux/2  "<Omega2>"
  Bus Selector6/1 -> Mux/1  "<Omega1>"
  Mux/1 -> Out1/1
  In1/1 -> Bus Selector6/1

== system CommercialVehicleLibrary2G/Utilities/To_workspace_truck_4axle/Subsystem4 ==
  In1 : Inport
  Bus Selector24 : BusSelector  OutputSignals=steeraxle1.Tire1_L.Fz,steeraxle1.Tire1_R.Fz,steeraxle2.Tire1_L.Fz,steeraxle2.Tire1_R.Fz,driveaxle1.Tire1_L.Fz,driveaxle1.Tire2_L.Fz,driveaxle1.Tire1_R.Fz,driveaxle1.Tire2_R.Fz,driveaxle2.Tire1_L.Fz,driveaxle2.Tire2_L.Fz,driveaxle2.Tire1_R.Fz,driveaxle2.Tire2_R.Fz
  Mux : Mux  Inputs=12
  Out1 : Outport
  wires:
  In1/1 -> Bus Selector24/1
  Mux/1 -> Out1/1
  Bus Selector24/5 -> Mux/5  "<Fz>"
  Bus Selector24/6 -> Mux/6  "<Fz>"
  Bus Selector24/7 -> Mux/7  "<Fz>"
  Bus Selector24/8 -> Mux/8  "<Fz>"
  Bus Selector24/9 -> Mux/9  "<Fz>"
  Bus Selector24/10 -> Mux/10  "<Fz>"
  Bus Selector24/11 -> Mux/11  "<Fz>"
  Bus Selector24/12 -> Mux/12  "<Fz>"
  Bus Selector24/1 -> Mux/1  "<Fz>"
  Bus Selector24/2 -> Mux/2  "<Fz>"
  Bus Selector24/3 -> Mux/3  "<Fz>"
  Bus Selector24/4 -> Mux/4  "<Fz>"

== system CommercialVehicleLibrary2G/Vehicles/Rigid Truck - 2 axles/Cameras ==
  Front Camera Transform : sm_lib/Frames and Transforms/Rigid Transform  TranslationMethod=Cartesian  TranslationStandardOffset=0  TranslationLengthUnit=m  TranslationStandardAxis=+Z  TranslationCartesianOffset=[-10 0 6]  TranslationROffset=0  TranslationROffsetUnits=m  TranslationZOffset=0  TranslationZOffsetUnits=m  TranslationThetaOffset=0  TranslationThetaOffsetUnits=deg  RotationMethod=None  RotationAngleUnits=deg  RotationStandardAxis=+Y  RotationAngle=90  RotationArbitraryAxis=[0 0 1]  FollAlignAxisA=+X  BaseAlignAxisA=+Y  FollAlignAxisB=+Y  BaseAlignAxisB=+Z  RotationSequenceAxes=FollowerAxes  RotationSequence=XYX  RotationSequenceAngles=[0 0 0]  RotationSequenceAnglesUnits=deg  RotationMatrix=[1 0 0; 0 1 0; 0 0 1]
  Side Camera Transform : sm_lib/Frames and Transforms/Rigid Transform  TranslationMethod=Cartesian  TranslationStandardOffset=0  TranslationLengthUnit=m  TranslationStandardAxis=+Z  TranslationCartesianOffset=[5 3 3]  TranslationROffset=0  TranslationROffsetUnits=m  TranslationZOffset=0  TranslationZOffsetUnits=m  TranslationThetaOffset=0  TranslationThetaOffsetUnits=deg  RotationMethod=None  RotationAngleUnits=deg  RotationStandardAxis=+Z  RotationAngle=90  RotationArbitraryAxis=[0 0 1]  FollAlignAxisA=+X  BaseAlignAxisA=+Y  FollAlignAxisB=+Y  BaseAlignAxisB=+Z  RotationSequenceAxes=FollowerAxes  RotationSequence=XYX  RotationSequenceAngles=[0 0 0]  RotationSequenceAnglesUnits=deg  RotationMatrix=[1 0 0; 0 1 0; 0 0 1]
  Spherical Solid : sm_lib/Body Elements/Spherical Solid  GraphicAmbientColor=[0.15 0.15 0.15 1.0]  BasedOnType=Density  CenterOfMass=[0 0 0]  CenterOfMassUnits=m  GraphicDiffuseColor=[0.5 0.5 0.5]  Density=1000  DensityUnits=kg/m^3  DoExposeReferenceFrame=on  GraphicEmissiveColor=[0.0 0.0 0.0 1.0]  ExportEntireGeometry=off  SerializedExposedGeometries=<ExposedGeometries/>  SerializedFrames=<Frames/>  MarkerShape=Sphere  MarkerSize=10  GraphicType=FromGeometry  InertiaType=PointMass  Mass=1e-09  MassUnits=kg  MomentsOfInertia=[1 1 1]  MomentsOfInertiaUnits=kg*m^2  GraphicOpacity=0  ProductsOfInertia=[0 0 0]  ProductsOfInertiaUnits=kg*m^2  GraphicShininess=75  GraphicSpecularColor=[0.5 0.5 0.5 1.0]  SphereRadius=1e-09  SphereRadiusUnits=m  GraphicVisPropType=SimpleVisualProperties
  Spherical Solid1 : sm_lib/Body Elements/Spherical Solid  GraphicAmbientColor=[0.15 0.15 0.15 1.0]  BasedOnType=Density  CenterOfMass=[0 0 0]  CenterOfMassUnits=m  GraphicDiffuseColor=[0.5 0.5 0.5]  Density=1000  DensityUnits=kg/m^3  DoExposeReferenceFrame=on  GraphicEmissiveColor=[0.0 0.0 0.0 1.0]  ExportEntireGeometry=off  SerializedExposedGeometries=<ExposedGeometries/>  SerializedFrames=<Frames/>  MarkerShape=Sphere  MarkerSize=10  GraphicType=FromGeometry  InertiaType=PointMass  Mass=1e-09  MassUnits=kg  MomentsOfInertia=[1 1 1]  MomentsOfInertiaUnits=kg*m^2  GraphicOpacity=0  ProductsOfInertia=[0 0 0]  ProductsOfInertiaUnits=kg*m^2  GraphicShininess=75  GraphicSpecularColor=[0.5 0.5 0.5 1.0]  SphereRadius=1e-09  SphereRadiusUnits=m  GraphicVisPropType=SimpleVisualProperties
  " " : PMIOPort  Side=Right
  connections:
  Side Camera Transform/LConn1 -- Front Camera Transform/LConn1 -- " "/RConn1
  Spherical Solid/RConn1 -- Side Camera Transform/RConn1
  Spherical Solid1/RConn1 -- Front Camera Transform/RConn1

== system CommercialVehicleLibrary2G/Vehicles/Rigid Truck - 2 axles/Measurements ==
  Bus Creator2 : BusCreator  Inputs=3
  Bus Creator3 : BusCreator  Inputs=3
  Fcn4 : Fcn  Expr=u(3)
  PS-Simulink Converter{3..8,10..11} (8 alike) : nesl_utility/PS-Simulink Converter  PhysicalDomain=network_engine_domain  SubClassName=ps_output  LeftPortType=input  RightPortType=output  PseudoPeriodic=off  Frequencies=[]  Unit=inherit  AffineConversion=off
  Scope : Scope
  Scope1 : Scope
  Transform Sensor1 : sm_lib/Frames and Transforms/Transform Sensor  MeasurementFrame=NonRotatingFollower  SenseAngle=off  SenseAxis=off  SenseAngle1=off  SenseAngle2=off  SenseAngle3=off  SenseQ=off  SenseR=off  SenseOmegaX=on  SenseOmegaY=on  SenseOmegaZ=on  SenseOmega1=off  SenseOmega2=off  SenseOmega3=off  SenseQDot=off  SenseRDot=off  SenseAlphaX=on  SenseAlphaY=on  SenseAlphaZ=on  SenseAlpha1=off  SenseAlpha2=off  SenseAlpha3=off  SenseQDDot=off  SenseRDDot=off  SenseX=off  SenseY=off  SenseZ=off  SenseRad=off  SenseAzim=off  SenseDist=off  SenseInc=off  SenseXDot=on  SenseYDot=on  SenseZDot=off  SenseRadDot=off  SenseAzimDot=off  SenseDistDot=off  SenseIncDot=off  SenseXDDot=off  SenseYDDot=off  SenseZDDot=off  SenseRadDDot=off  SenseAzimDDot=off  SenseDistDDot=off  SenseIncDDot=off
  Transform Sensor2 : PMIOPort  Side=Left
  Transform Sensor3 : PMIOPort  Port=2  Side=Right
  Out1 : Outport
  Out2 : Outport  Port=2
  Out3 : Outport  Port=3
  wires:
  PS-Simulink Converter3/1 -> Bus Creator2/3
  PS-Simulink Converter5/1 -> Bus Creator2/1
  PS-Simulink Converter10/1 -> Scope1/1
  PS-Simulink Converter7/1 -> Bus Creator3/2
  Bus Creator2/1 -> Fcn4/1
  PS-Simulink Converter8/1 -> Bus Creator3/1
  Bus Creator3/1 -> Out2/1
  PS-Simulink Converter6/1 -> Bus Creator3/3
  PS-Simulink Converter4/1 -> Bus Creator2/2
  Fcn4/1 -> Out1/1
  PS-Simulink Converter11/1 -> Out3/1, Scope/1
  connections:
  PS-Simulink Converter11/LConn1 -- Transform Sensor1/RConn8
  PS-Simulink Converter7/LConn1 -- Transform Sensor1/RConn6
  Transform Sensor1/RConn2 -- PS-Simulink Converter5/LConn1
  PS-Simulink Converter6/LConn1 -- Transform Sensor1/RConn7
  PS-Simulink Converter3/LConn1 -- Transform Sensor1/RConn4
  Transform Sensor1/RConn1 -- Transform Sensor3/RConn1
  PS-Simulink Converter8/LConn1 -- Transform Sensor1/RConn5
  PS-Simulink Converter4/LConn1 -- Transform Sensor1/RConn3
  Transform Sensor1/RConn9 -- PS-Simulink Converter10/LConn1
  Transform Sensor1/LConn1 -- Transform Sensor2/RConn1

== system CommercialVehicleLibrary2G/Vehicles/Rigid Truck - 3 axles/Cameras ==
  Front Camera Transform : sm_lib/Frames and Transforms/Rigid Transform  TranslationMethod=Cartesian  TranslationStandardOffset=0  TranslationLengthUnit=m  TranslationStandardAxis=+Z  TranslationCartesianOffset=[-10 0 6]  TranslationROffset=0  TranslationROffsetUnits=m  TranslationZOffset=0  TranslationZOffsetUnits=m  TranslationThetaOffset=0  TranslationThetaOffsetUnits=deg  RotationMethod=None  RotationAngleUnits=deg  RotationStandardAxis=+Y  RotationAngle=90  RotationArbitraryAxis=[0 0 1]  FollAlignAxisA=+X  BaseAlignAxisA=+Y  FollAlignAxisB=+Y  BaseAlignAxisB=+Z  RotationSequenceAxes=FollowerAxes  RotationSequence=XYX  RotationSequenceAngles=[0 0 0]  RotationSequenceAnglesUnits=deg  RotationMatrix=[1 0 0; 0 1 0; 0 0 1]
  Side Camera Transform : sm_lib/Frames and Transforms/Rigid Transform  TranslationMethod=Cartesian  TranslationStandardOffset=0  TranslationLengthUnit=m  TranslationStandardAxis=+Z  TranslationCartesianOffset=[5 3 3]  TranslationROffset=0  TranslationROffsetUnits=m  TranslationZOffset=0  TranslationZOffsetUnits=m  TranslationThetaOffset=0  TranslationThetaOffsetUnits=deg  RotationMethod=None  RotationAngleUnits=deg  RotationStandardAxis=+Z  RotationAngle=90  RotationArbitraryAxis=[0 0 1]  FollAlignAxisA=+X  BaseAlignAxisA=+Y  FollAlignAxisB=+Y  BaseAlignAxisB=+Z  RotationSequenceAxes=FollowerAxes  RotationSequence=XYX  RotationSequenceAngles=[0 0 0]  RotationSequenceAnglesUnits=deg  RotationMatrix=[1 0 0; 0 1 0; 0 0 1]
  Spherical Solid : sm_lib/Body Elements/Spherical Solid  GraphicAmbientColor=[0.15 0.15 0.15 1.0]  BasedOnType=Density  CenterOfMass=[0 0 0]  CenterOfMassUnits=m  GraphicDiffuseColor=[0.5 0.5 0.5]  Density=1000  DensityUnits=kg/m^3  DoExposeReferenceFrame=on  GraphicEmissiveColor=[0.0 0.0 0.0 1.0]  ExportEntireGeometry=off  SerializedExposedGeometries=<ExposedGeometries/>  SerializedFrames=<Frames/>  MarkerShape=Sphere  MarkerSize=10  GraphicType=FromGeometry  InertiaType=PointMass  Mass=1e-09  MassUnits=kg  MomentsOfInertia=[1 1 1]  MomentsOfInertiaUnits=kg*m^2  GraphicOpacity=0  ProductsOfInertia=[0 0 0]  ProductsOfInertiaUnits=kg*m^2  GraphicShininess=75  GraphicSpecularColor=[0.5 0.5 0.5 1.0]  SphereRadius=1e-09  SphereRadiusUnits=m  GraphicVisPropType=SimpleVisualProperties
  Spherical Solid1 : sm_lib/Body Elements/Spherical Solid  GraphicAmbientColor=[0.15 0.15 0.15 1.0]  BasedOnType=Density  CenterOfMass=[0 0 0]  CenterOfMassUnits=m  GraphicDiffuseColor=[0.5 0.5 0.5]  Density=1000  DensityUnits=kg/m^3  DoExposeReferenceFrame=on  GraphicEmissiveColor=[0.0 0.0 0.0 1.0]  ExportEntireGeometry=off  SerializedExposedGeometries=<ExposedGeometries/>  SerializedFrames=<Frames/>  MarkerShape=Sphere  MarkerSize=10  GraphicType=FromGeometry  InertiaType=PointMass  Mass=1e-09  MassUnits=kg  MomentsOfInertia=[1 1 1]  MomentsOfInertiaUnits=kg*m^2  GraphicOpacity=0  ProductsOfInertia=[0 0 0]  ProductsOfInertiaUnits=kg*m^2  GraphicShininess=75  GraphicSpecularColor=[0.5 0.5 0.5 1.0]  SphereRadius=1e-09  SphereRadiusUnits=m  GraphicVisPropType=SimpleVisualProperties
  " " : PMIOPort  Side=Right
  connections:
  Side Camera Transform/LConn1 -- Front Camera Transform/LConn1 -- " "/RConn1
  Spherical Solid/RConn1 -- Side Camera Transform/RConn1
  Spherical Solid1/RConn1 -- Front Camera Transform/RConn1

== system CommercialVehicleLibrary2G/Vehicles/Rigid Truck - 3 axles/Measurements ==
  Bus Creator2 : BusCreator  Inputs=3
  Bus Creator3 : BusCreator  Inputs=3
  Fcn4 : Fcn  Expr=u(3)
  PS-Simulink Converter{3..8,10..11} (8 alike) : nesl_utility/PS-Simulink Converter  PhysicalDomain=network_engine_domain  SubClassName=ps_output  LeftPortType=input  RightPortType=output  PseudoPeriodic=off  Frequencies=[]  Unit=inherit  AffineConversion=off
  Scope : Scope
  Scope1 : Scope
  Transform Sensor1 : sm_lib/Frames and Transforms/Transform Sensor  MeasurementFrame=NonRotatingFollower  SenseAngle=off  SenseAxis=off  SenseAngle1=off  SenseAngle2=off  SenseAngle3=off  SenseQ=off  SenseR=off  SenseOmegaX=on  SenseOmegaY=on  SenseOmegaZ=on  SenseOmega1=off  SenseOmega2=off  SenseOmega3=off  SenseQDot=off  SenseRDot=off  SenseAlphaX=on  SenseAlphaY=on  SenseAlphaZ=on  SenseAlpha1=off  SenseAlpha2=off  SenseAlpha3=off  SenseQDDot=off  SenseRDDot=off  SenseX=off  SenseY=off  SenseZ=off  SenseRad=off  SenseAzim=off  SenseDist=off  SenseInc=off  SenseXDot=on  SenseYDot=on  SenseZDot=off  SenseRadDot=off  SenseAzimDot=off  SenseDistDot=off  SenseIncDot=off  SenseXDDot=off  SenseYDDot=off  SenseZDDot=off  SenseRadDDot=off  SenseAzimDDot=off  SenseDistDDot=off  SenseIncDDot=off
  Transform Sensor2 : PMIOPort  Side=Left
  Transform Sensor3 : PMIOPort  Port=2  Side=Right
  Out1 : Outport
  Out2 : Outport  Port=2
  Out3 : Outport  Port=3
  wires:
  PS-Simulink Converter3/1 -> Bus Creator2/3
  PS-Simulink Converter5/1 -> Bus Creator2/1
  PS-Simulink Converter10/1 -> Scope1/1
  PS-Simulink Converter7/1 -> Bus Creator3/2
  Bus Creator2/1 -> Fcn4/1
  PS-Simulink Converter8/1 -> Bus Creator3/1
  Bus Creator3/1 -> Out2/1
  PS-Simulink Converter6/1 -> Bus Creator3/3
  PS-Simulink Converter4/1 -> Bus Creator2/2
  Fcn4/1 -> Out1/1
  PS-Simulink Converter11/1 -> Out3/1, Scope/1
  connections:
  PS-Simulink Converter11/LConn1 -- Transform Sensor1/RConn8
  PS-Simulink Converter7/LConn1 -- Transform Sensor1/RConn6
  Transform Sensor1/RConn2 -- PS-Simulink Converter5/LConn1
  PS-Simulink Converter6/LConn1 -- Transform Sensor1/RConn7
  PS-Simulink Converter3/LConn1 -- Transform Sensor1/RConn4
  Transform Sensor1/RConn1 -- Transform Sensor3/RConn1
  PS-Simulink Converter8/LConn1 -- Transform Sensor1/RConn5
  PS-Simulink Converter4/LConn1 -- Transform Sensor1/RConn3
  Transform Sensor1/RConn9 -- PS-Simulink Converter10/LConn1
  Transform Sensor1/LConn1 -- Transform Sensor2/RConn1

== system CommercialVehicleLibrary2G/Vehicles/Rigid Truck - 4 axles/Cameras ==
  Front Camera Transform : sm_lib/Frames and Transforms/Rigid Transform  TranslationMethod=Cartesian  TranslationStandardOffset=0  TranslationLengthUnit=m  TranslationStandardAxis=+Z  TranslationCartesianOffset=[-10 0 6]  TranslationROffset=0  TranslationROffsetUnits=m  TranslationZOffset=0  TranslationZOffsetUnits=m  TranslationThetaOffset=0  TranslationThetaOffsetUnits=deg  RotationMethod=None  RotationAngleUnits=deg  RotationStandardAxis=+Y  RotationAngle=90  RotationArbitraryAxis=[0 0 1]  FollAlignAxisA=+X  BaseAlignAxisA=+Y  FollAlignAxisB=+Y  BaseAlignAxisB=+Z  RotationSequenceAxes=FollowerAxes  RotationSequence=XYX  RotationSequenceAngles=[0 0 0]  RotationSequenceAnglesUnits=deg  RotationMatrix=[1 0 0; 0 1 0; 0 0 1]
  Side Camera Transform : sm_lib/Frames and Transforms/Rigid Transform  TranslationMethod=Cartesian  TranslationStandardOffset=0  TranslationLengthUnit=m  TranslationStandardAxis=+Z  TranslationCartesianOffset=[5 3 3]  TranslationROffset=0  TranslationROffsetUnits=m  TranslationZOffset=0  TranslationZOffsetUnits=m  TranslationThetaOffset=0  TranslationThetaOffsetUnits=deg  RotationMethod=None  RotationAngleUnits=deg  RotationStandardAxis=+Z  RotationAngle=90  RotationArbitraryAxis=[0 0 1]  FollAlignAxisA=+X  BaseAlignAxisA=+Y  FollAlignAxisB=+Y  BaseAlignAxisB=+Z  RotationSequenceAxes=FollowerAxes  RotationSequence=XYX  RotationSequenceAngles=[0 0 0]  RotationSequenceAnglesUnits=deg  RotationMatrix=[1 0 0; 0 1 0; 0 0 1]
  Spherical Solid : sm_lib/Body Elements/Spherical Solid  GraphicAmbientColor=[0.15 0.15 0.15 1.0]  BasedOnType=Density  CenterOfMass=[0 0 0]  CenterOfMassUnits=m  GraphicDiffuseColor=[0.5 0.5 0.5]  Density=1000  DensityUnits=kg/m^3  DoExposeReferenceFrame=on  GraphicEmissiveColor=[0.0 0.0 0.0 1.0]  ExportEntireGeometry=off  SerializedExposedGeometries=<ExposedGeometries/>  SerializedFrames=<Frames/>  MarkerShape=Sphere  MarkerSize=10  GraphicType=FromGeometry  InertiaType=PointMass  Mass=1e-09  MassUnits=kg  MomentsOfInertia=[1 1 1]  MomentsOfInertiaUnits=kg*m^2  GraphicOpacity=0  ProductsOfInertia=[0 0 0]  ProductsOfInertiaUnits=kg*m^2  GraphicShininess=75  GraphicSpecularColor=[0.5 0.5 0.5 1.0]  SphereRadius=1e-09  SphereRadiusUnits=m  GraphicVisPropType=SimpleVisualProperties
  Spherical Solid1 : sm_lib/Body Elements/Spherical Solid  GraphicAmbientColor=[0.15 0.15 0.15 1.0]  BasedOnType=Density  CenterOfMass=[0 0 0]  CenterOfMassUnits=m  GraphicDiffuseColor=[0.5 0.5 0.5]  Density=1000  DensityUnits=kg/m^3  DoExposeReferenceFrame=on  GraphicEmissiveColor=[0.0 0.0 0.0 1.0]  ExportEntireGeometry=off  SerializedExposedGeometries=<ExposedGeometries/>  SerializedFrames=<Frames/>  MarkerShape=Sphere  MarkerSize=10  GraphicType=FromGeometry  InertiaType=PointMass  Mass=1e-09  MassUnits=kg  MomentsOfInertia=[1 1 1]  MomentsOfInertiaUnits=kg*m^2  GraphicOpacity=0  ProductsOfInertia=[0 0 0]  ProductsOfInertiaUnits=kg*m^2  GraphicShininess=75  GraphicSpecularColor=[0.5 0.5 0.5 1.0]  SphereRadius=1e-09  SphereRadiusUnits=m  GraphicVisPropType=SimpleVisualProperties
  " " : PMIOPort  Side=Right
  connections:
  Side Camera Transform/LConn1 -- Front Camera Transform/LConn1 -- " "/RConn1
  Spherical Solid/RConn1 -- Side Camera Transform/RConn1
  Spherical Solid1/RConn1 -- Front Camera Transform/RConn1
